simulink model "ITACG_3D_salvo_simulation"  (R2023b)
settings: Solver=ode4  StartTime=0.0  StopTime=28  FixedStep=1/10  RelTol=1e-3
libraries: simulink_extras x40, simulink x4
(part 2 of 2)

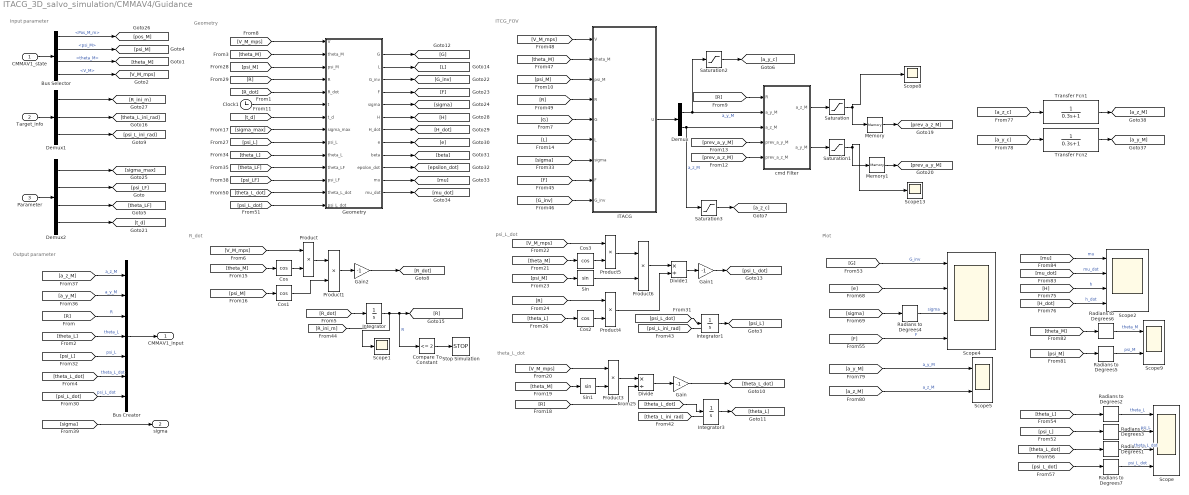
== system ITACG_3D_salvo_simulation/CMMAV4/Guidance ==
  note: Input parameter
  note: ITCG_FOV
  note: R_dot
  note: psi_L_dot
  note: theta_L_dot
  note: Output parameter
  note: Geometry
  note: Plot
  CMMAV1_state : Inport
  Target_info : Inport  Port=2
  Parameter : Inport  Port=3
  Bus Creator : BusCreator  Inputs=7
  Bus Selector : BusSelector  OutputSignals=Pos_M_m,psi_M,theta_M,V_M
  Clock1 : Clock
  Compare To Constant : simulink/Logic and Bit Operations/Compare To Constant  relop=<=  const=2  OutDataTypeStr=boolean
  Cos{,1..3} (4 alike) : Trigonometry  Operator=cos
  Demux : Demux  Outputs=2
  Demux1 : Demux  Outputs=3
  Demux2 : Demux
  Divide : Product  Inputs=*/
  Divide1 : Product  Inputs=*/
  Gain : Gain  Gain=-1
  Gain1 : Gain  Gain=-1
  Gain2 : Gain  Gain=-1
  Geometry : MATLAB Function  TreatAsAtomicUnit=on
  ITACG : MATLAB Function  TreatAsAtomicUnit=on
  Integrator : Integrator  InitialCondition=700
  Integrator1 : Integrator  InitialCondition=10*pi/180
  Integrator3 : Integrator  InitialCondition=-40*pi/180
  Memory : Memory
  Memory1 : Memory
  Product{,1,3..6} (6 alike) : Product
  Radians to Degrees{1..7} (7 alike) : simulink_extras/Transformations/Radians to Degrees
  Saturation{,1..3} (4 alike) : Saturate  UpperLimit=100  LowerLimit=-100
  Scope : Scope  NumInputPorts=4
  Scope1 : Scope
  Scope13 : Scope
  Scope2 : Scope  NumInputPorts=4
  Scope4 : Scope  NumInputPorts=4
  Scope5 : Scope  NumInputPorts=2
  Scope8 : Scope
  Scope9 : Scope  NumInputPorts=2
  Sin : Trigonometry
  Sin1 : Trigonometry
  Stop Simulation : Stop
  Transfer Fcn1 : TransferFcn  Denominator=[0.3 1]  ParameterTunability=Optimized
  Transfer Fcn2 : TransferFcn  Denominator=[0.3 1]  ParameterTunability=Optimized
  cmd Filter : MATLAB Function  TreatAsAtomicUnit=on
  CMMAV1_input : Outport
  sigma : Outport  Port=2
  wires:
  Product1/1 -> Gain2/1
  Gain2/1 -> [R_dot]
  [theta_L] -> Cos2/1
  [theta_L_dot] -> Integrator3/1
  Gain/1 -> [theta_L_dot]
  Product5/1 -> Product6/1
  Divide1/1 -> Gain1/1
  [V_M_mps] -> Product3/1
  [V_M_mps] -> Product5/1
  [theta_M] -> Sin1/1
  [R] -> Divide/2
  [theta_M] -> Cos3/1
  Divide/1 -> Gain/1
  [theta_M] -> Cos/1
  [R] -> Product4/1
  Product4/1 -> Divide1/2
  Integrator3/1 -> [theta_L]
  [psi_L_dot] -> Integrator1/1
  Sin1/1 -> Product3/2
  Product3/1 -> Divide/1
  [psi_M] -> Cos1/1
  Cos/1 -> Product/2
  Integrator1/1 -> [psi_L]
  Product6/1 -> Divide1/1
  [psi_M] -> Sin/1
  Compare To Constant/1 -> Stop Simulation/1
  [V_M_mps] -> Product/1
  Cos3/1 -> Product5/2
  Sin/1 -> Product6/2
  Integrator/1 -> Scope1/1, [R], Compare To Constant/1  "R"
  Product/1 -> Product1/1
  Cos2/1 -> Product4/2
  Cos1/1 -> Product1/2
  Gain1/1 -> [psi_L_dot]
  [R_dot] -> Integrator/1
  CMMAV1_state/1 -> Bus Selector/1
  Target_info/1 -> Demux1/1
  Demux2/1 -> [sigma_max]
  Parameter/1 -> Demux2/1
  Bus Selector/1 -> [pos_M]  "<Pos_M_m>"
  Bus Selector/4 -> [V_M_mps]  "<V_M>"
  Demux1/2 -> [theta_L_ini_rad]
  Demux1/3 -> [psi_L_ini_rad]
  Demux1/1 -> [R_ini_m]
  [psi_L] -> Bus Creator/5  "psi_L"
  [theta_L] -> Bus Creator/4  "theta_L"
  Bus Creator/1 -> CMMAV1_input/1
  [a_y_M] -> Bus Creator/2  "a_y_M"
  [R] -> Bus Creator/3  "R"
  [a_z_M] -> Bus Creator/1  "a_z_M"
  [theta_L_ini_rad] -> ?
  [psi_L_ini_rad] -> ?
  [R_ini_m] -> ?
  Bus Selector/2 -> [psi_M]  "<psi_M>"
  Bus Selector/3 -> [theta_M]  "<theta_M>"
  [psi_M] -> Geometry/3(psi_M)
  [V_M_mps] -> Geometry/1(V)
  [theta_M] -> Geometry/2(theta_M)
  [R] -> Geometry/4(R)
  Demux2/2 -> [psi_LF]
  Demux2/3 -> [theta_LF]
  Demux2/4 -> [t_d]
  Saturation2/1 -> [a_y_c]
  Saturation3/1 -> [a_z_c]
  cmd Filter/1(a_z_M) -> Saturation/1
  Memory/1 -> [prev_a_z_M]
  Transfer Fcn2/1 -> [a_y_M]
  Transfer Fcn1/1 -> [a_z_M]
  cmd Filter/2(a_y_M) -> Saturation1/1
  Saturation1/1 -> Scope13/1, Memory1/1
  Saturation/1 -> Scope8/1, Memory/1
  Demux/2 -> cmd Filter/3("a_z_M "), Saturation3/1  "a_z_M"
  [prev_a_y_M] -> cmd Filter/4(prev_a_y_M)
  [prev_a_z_M] -> cmd Filter/5(prev_a_z_M)
  [a_z_c] -> Transfer Fcn1/1
  Demux/1 -> cmd Filter/2("a_y_M "), Saturation2/1  "a_y_M"
  Memory1/1 -> [prev_a_y_M]
  [a_y_c] -> Transfer Fcn2/1
  [R] -> cmd Filter/1(R)
  ITACG/1(U) -> Demux/1
  [theta_LF] -> Geometry/11(theta_LF)
  [psi_LF] -> Geometry/12(psi_LF)
  [theta_L_dot] -> Geometry/13(theta_L_dot)
  [R_dot] -> Geometry/5(R_dot)
  [t_d] -> Geometry/7(t_d)
  [sigma_max] -> Geometry/8(sigma_max)
  [psi_L] -> Geometry/9(psi_L)
  [theta_L] -> Geometry/10(theta_L)
  [psi_L_dot] -> Geometry/14(psi_L_dot)
  Clock1/1 -> Geometry/6(t)
  Geometry/1(G) -> [G]
  Geometry/2(L) -> [L]
  Geometry/3(G_inv) -> [G_inv]
  Geometry/4(F) -> [F]
  Geometry/5(sigma) -> [sigma]
  Geometry/6(H) -> [H]
  Geometry/7(H_dot) -> [H_dot]
  Geometry/8(e) -> [e]
  Geometry/9(beta) -> [beta]
  Geometry/10(epsilon_dot) -> [epsilon_dot]
  Geometry/11(mu) -> [mu]
  Geometry/12(mu_dot) -> [mu_dot]
  [V_M_mps] -> ITACG/1(V)
  [theta_M] -> ITACG/2(theta_M)
  [psi_M] -> ITACG/3(psi_M)
  [G] -> ITACG/5(G)
  [L] -> ITACG/6(L)
  [sigma] -> ITACG/7(sigma)
  [F] -> ITACG/8(F)
  [G_inv] -> ITACG/9(G_inv)
  [R] -> ITACG/4(R)
  Radians to Degrees6/1 -> Scope9/1  "theta_M"
  Radians to Degrees7/1 -> Scope/4  "psi_L_dot"
  [psi_M] -> Radians to Degrees5/1
  [theta_L_dot] -> Radians to Degrees1/1
  Radians to Degrees3/1 -> Scope/2  "psi_L"
  [theta_L] -> Radians to Degrees2/1
  Radians to Degrees4/1 -> Scope4/3  "sigma"
  Radians to Degrees2/1 -> Scope/1  "theta_L"
  Radians to Degrees5/1 -> Scope9/2  "psi_M"
  [H] -> Scope2/3  "h"
  [psi_L] -> Radians to Degrees3/1
  [mu] -> Scope2/1  "mu"
  [mu_dot] -> Scope2/2  "mu_dot"
  Radians to Degrees1/1 -> Scope/3  "theta_L_dot"
  [sigma] -> Radians to Degrees4/1
  [a_y_M] -> Scope5/1  "a_y_M"
  [a_z_M] -> Scope5/2  "a_z_M"
  [G] -> Scope4/1  "G_inv"
  [theta_M] -> Radians to Degrees6/1
  [psi_L_dot] -> Radians to Degrees7/1
  [F] -> Scope4/4  "F"
  [H_dot] -> Scope2/4  "h_dot"
  [e] -> Scope4/2
  [theta_L_dot] -> Bus Creator/6  "theta_L_dot"
  [psi_L_dot] -> Bus Creator/7  "psi_L_dot"
  [sigma] -> sigma/1

== system ITACG_3D_salvo_simulation/CMMAV4/Parameter init ==
  Constant : Constant  Value=45
  Constant1 : Constant  Value=0
  Constant2 : Constant  Value=-80
  Constant3 : Constant  Value=28
  Degrees to Radians : simulink_extras/Transformations/Degrees to Radians
  Degrees to Radians1 : simulink_extras/Transformations/Degrees to Radians
  Degrees to Radians2 : simulink_extras/Transformations/Degrees to Radians
  Mux : Mux
  Parameter : Outport
  wires:
  Mux/1 -> Parameter/1
  Constant3/1 -> Mux/4  "t_d"
  Constant2/1 -> Degrees to Radians2/1
  Constant1/1 -> Degrees to Radians1/1
  Constant/1 -> Degrees to Radians/1
  Degrees to Radians2/1 -> Mux/3  "theta_LF"
  Degrees to Radians1/1 -> Mux/2  "psi_LF"
  Degrees to Radians/1 -> Mux/1  "sigma_max"

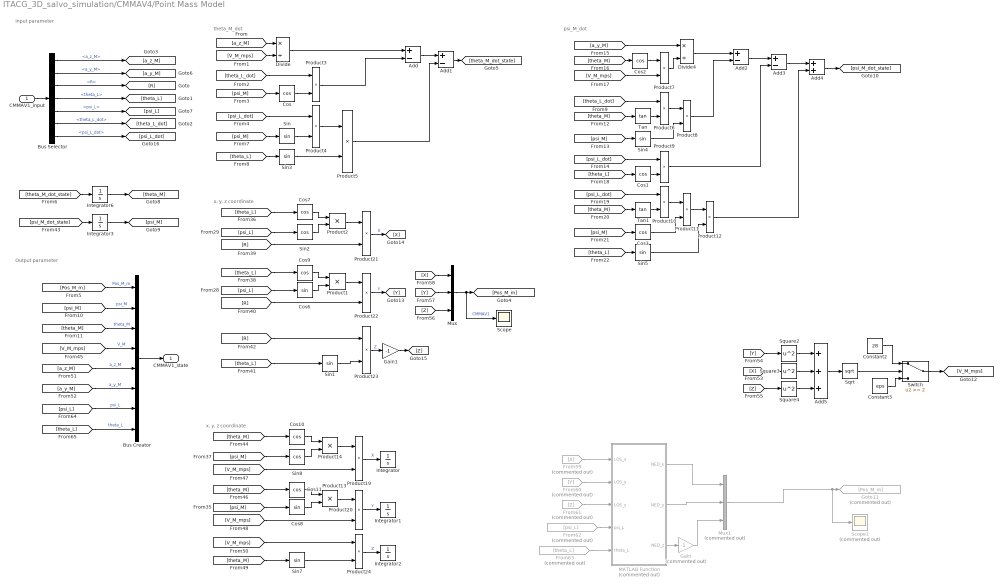
== system ITACG_3D_salvo_simulation/CMMAV4/Point Mass Model ==
  note: Input parameter
  note: x, y, z coordinate
  note: Output parameter
  note: x, y, z coordinate
  note: theta_M_dot
  note: psi_M_dot
  CMMAV1_input : Inport
  Add{,1..3} (4 alike) : Sum  Inputs=+-
  Add4 : Sum
  Add5 : Sum  Inputs=+++
  Bus Creator : BusCreator  Inputs=8
  Bus Selector : BusSelector  OutputSignals=a_z_M,a_y_M,R,theta_L,psi_L,theta_L_dot,psi_L_dot
  Constant2 : Constant  Value=28
  Constant3 : Constant  Value=eps
  Cos{,1..3,7,9..11} (8 alike) : Trigonometry  Operator=cos
  Cos6 : Trigonometry
  Cos8 : Trigonometry
  Divide : Product  Inputs=*/
  Divide4 : Product  Inputs=*/
  From59 : From  Commented=on  GotoTag=X
  From60 : From  Commented=on  GotoTag=Y
  From61 : From  Commented=on  GotoTag=Z
  From62 : From  Commented=on  GotoTag=psi_L
  From63 : From  Commented=on  GotoTag=theta_L
  Gain : Gain  Commented=on  Gain=-1
  Gain1 : Gain  Gain=-1
  Goto11 : Goto  Commented=on  GotoTag=Pos_M_m
  Integrator : Integrator
  Integrator1 : Integrator
  Integrator2 : Integrator
  Integrator3 : Integrator  InitialCondition=10*pi/180
  Integrator6 : Integrator  InitialCondition=10*pi/180
  MATLAB Function : MATLAB Function  Commented=on  TreatAsAtomicUnit=on
  Mux : Mux  Inputs=3
  Mux1 : Mux  Commented=on  Inputs=3
  Product{1..14,19..24} (20 alike) : Product
  Scope : Scope
  Scope1 : Scope  Commented=on
  Sin{,1,3..5,7} (6 alike) : Trigonometry
  Sin2 : Trigonometry  Operator=cos
  Sin8 : Trigonometry  Operator=cos
  Sqrt : Sqrt
  Square2 : Math  Operator=square
  Square3 : Math  Operator=square
  Square4 : Math  Operator=square
  Switch : Switch  Threshold=2  SaturateOnIntegerOverflow=off  InputSameDT=off
  Tan : Trigonometry  Operator=tan
  Tan1 : Trigonometry  Operator=tan
  CMMAV1_state : Outport
  wires:
  [psi_M] -> Bus Creator/2  "psi_M"
  [psi_M_dot_state] -> Integrator3/1
  [theta_L] -> Cos9/1
  [V_M_mps] -> Bus Creator/4  "V_M"
  Cos6/1 -> Product1/2
  Bus Selector/2 -> [a_y_M]  "<a_y_M>"
  Integrator6/1 -> [theta_M]
  [psi_L] -> Cos6/1
  Bus Selector/5 -> [psi_L]  "<psi_L>"
  Product21/1 -> [X]  "X"
  Product1/1 -> Product22/1
  Integrator3/1 -> [psi_M]
  Sin2/1 -> Product2/2
  Bus Selector/1 -> [a_z_M]  "<a_z_M>"
  Mux/1 -> [Pos_M_m], Scope/1  "CMMAV1"
  Bus Selector/3 -> [R]  "<R>"
  [theta_M] -> Bus Creator/3  "theta_M"
  [psi_L] -> Sin2/1
  Product2/1 -> Product21/1
  Cos9/1 -> Product1/1
  [theta_L] -> Cos7/1
  Cos7/1 -> Product2/1
  [theta_M_dot_state] -> Integrator6/1
  Product22/1 -> [Y]  "Y"
  [V_M_mps] -> Product24/1
  Sin7/1 -> Product24/2
  [V_M_mps] -> Product20/2
  [theta_M] -> Cos11/1
  [psi_M] -> Sin8/1
  [theta_M] -> Sin7/1
  Sin8/1 -> Product14/2
  Product14/1 -> Product19/1
  Product19/1 -> Integrator/1  "X"
  Product13/1 -> Product20/1
  Product24/1 -> Integrator2/1  "Z"
  [psi_M] -> Cos8/1
  [V_M_mps] -> Product19/2
  [theta_M] -> Cos10/1
  Cos11/1 -> Product13/1
  Cos8/1 -> Product13/2
  Product20/1 -> Integrator1/1  "Y"
  Cos10/1 -> Product14/1
  [R] -> Product21/2
  [R] -> Product22/2
  [R] -> Product23/1
  Sin1/1 -> Product23/2
  [theta_L] -> Sin1/1
  CMMAV1_input/1 -> Bus Selector/1
  [Pos_M_m] -> Bus Creator/1  "Pos_M_m"
  Bus Creator/1 -> CMMAV1_state/1
  Bus Selector/4 -> [theta_L]  "<theta_L>"
  [a_z_M] -> Bus Creator/5  "a_z_M"
  [a_y_M] -> Bus Creator/6  "a_y_M"
  Constant3/1 -> Switch/3
  Switch/1 -> [V_M_mps]
  Sqrt/1 -> Switch/2
  Add5/1 -> Sqrt/1
  Square2/1 -> Add5/1
  [Y] -> Square2/1
  Constant2/1 -> Switch/1
  [X] -> Square3/1
  Square3/1 -> Add5/2
  Product23/1 -> Gain1/1  "Z"
  [Z] -> Square4/1
  [X] -> Mux/1
  [Y] -> Mux/2
  [Z] -> Mux/3
  Square4/1 -> Add5/3
  From59/1 -> MATLAB Function/1(LOS_x)
  From60/1 -> MATLAB Function/2(LOS_y)
  From61/1 -> MATLAB Function/3(LOS_z)
  From62/1 -> MATLAB Function/4(psi_L)
  From63/1 -> MATLAB Function/5(theta_L)
  MATLAB Function/2(NED_y) -> Mux1/2
  MATLAB Function/1(NED_x) -> Mux1/1
  MATLAB Function/3(NED_z) -> Gain/1
  Gain/1 -> Mux1/3
  Mux1/1 -> Scope1/1, Goto11/1
  [psi_L] -> Bus Creator/7  "psi_L"
  [theta_L] -> Bus Creator/8  "theta_L"
  Product5/1 -> Add1/2
  Add/1 -> Add1/1
  Product4/1 -> Product5/1
  [a_z_M] -> Divide/1
  Divide/1 -> Add/1
  [V_M_mps] -> Divide/2
  Sin3/1 -> Product5/2
  Sin/1 -> Product4/2
  [psi_L_dot] -> Product4/1
  [psi_M] -> Cos/1
  Cos/1 -> Product3/2
  Add1/1 -> [theta_M_dot_state]
  Product3/1 -> Add/2
  [psi_M] -> Sin/1
  [theta_L] -> Sin3/1
  [theta_L_dot] -> Product3/1
  Product8/1 -> Add2/2
  [a_y_M] -> Divide4/1
  Product7/1 -> Divide4/2
  Divide4/1 -> Add2/1
  [V_M_mps] -> Product7/2
  Product6/1 -> Product8/1
  Product10/1 -> Product11/1
  Tan1/1 -> Product10/2
  [theta_L] -> Cos1/1
  Product12/1 -> Add4/2
  [theta_L] -> Sin5/1
  Product11/1 -> Product12/1
  [theta_L_dot] -> Product6/1
  Sin5/1 -> Product12/2
  Cos3/1 -> Product11/2
  [psi_M] -> Cos3/1
  Product9/1 -> Add3/2
  Add4/1 -> [psi_M_dot_state]
  [psi_L_dot] -> Product10/1
  [theta_M] -> Tan1/1
  Cos1/1 -> Product9/2
  [theta_M] -> Cos2/1
  Sin4/1 -> Product8/2
  [psi_M] -> Sin4/1
  [theta_M] -> Tan/1
  Tan/1 -> Product6/2
  [psi_L_dot] -> Product9/1
  Cos2/1 -> Product7/1
  Add2/1 -> Add3/1
  Add3/1 -> Add4/1
  Gain1/1 -> [Z]
  Bus Selector/6 -> [theta_L_dot]  "<theta_L_dot>"
  Bus Selector/7 -> [psi_L_dot]  "<psi_L_dot>"

== system ITACG_3D_salvo_simulation/CMMAV4/Target ==
  note: LOS_angle initial
  note: Target position
  note: Target parameter
  note: Output parameter
  note: R_initial
  note: Output parameter
  Add : Sum
  Add1 : Sum
  Add2 : Sum
  Asin : Trigonometry  Operator=asin
  Asin1 : Trigonometry  Operator=acos
  Demux : Demux  Outputs=3
  Demux1 : Demux  Outputs=3
  Divide : Product  Inputs=*/
  Divide1 : Product  Inputs=*/
  Integrator : Integrator
  Integrator1 : Integrator
  Integrator2 : Integrator
  Mux : Mux  Inputs=3
  Mux1 : Mux  Inputs=3
  Scope : Scope
  Sqrt : Sqrt
  Sqrt1 : Sqrt
  Square{1..5} (5 alike) : Math  Operator=square
  Sum : Sum  Inputs=+++
  Sum1 : Sum  Inputs=++|
  Target Position : Constant  Value=[300;-500;300]  VectorParams1D=off
  Target Velocity : Constant  Value=[0;0;0]  VectorParams1D=off
  Target_info : Outport
  wires:
  [psi_L_ini_rad] -> Mux/3
  Asin/1 -> [theta_L_ini_rad]
  [rT_ini_z_m] -> Mux1/3
  [rM_z] -> Add2/1
  Demux/3 -> [vT_z]
  [vT_z] -> Integrator2/1
  Demux/2 -> [vT_y]
  [rT_ini_x_m] -> Mux1/1
  Add1/1 -> [rT_ini_y_m]  "Y"
  Square2/1 -> Sum/1
  [vT_x] -> Integrator/1
  Mux1/1 -> [Pos_T_m]
  Square3/1 -> Sum/2
  Add2/1 -> [rT_ini_z_m]  "Z"
  Integrator/1 -> [vT_xt]
  Sum/1 -> Sqrt/1
  Demux1/3 -> [rM_z]
  [rT_ini_y_m] -> Mux1/2
  Integrator1/1 -> [vT_yt]
  Demux/1 -> [vT_x]
  Demux1/1 -> [rM_x]
  Target Velocity/1 -> Demux/1
  Demux1/2 -> [rM_y]
  Add/1 -> [rT_ini_x_m]  "X"
  [vT_yt] -> Add1/2
  Divide1/1 -> Asin1/1
  [rM_x] -> Add/1
  [vT_zt] -> Add2/2
  Sum1/1 -> Sqrt1/1
  [rT_ini_x_m] -> Square1/1
  Square1/1 -> Sum1/1
  Square5/1 -> Sum1/2
  [rT_ini_y_m] -> Square5/1
  [vT_y] -> Integrator1/1
  [rM_y] -> Add1/1
  [rT_ini_z_m] -> Divide/1
  [R_ini_m] -> Mux/1
  Sqrt/1 -> Scope/1, [R_ini_m]
  [R_ini_m] -> Divide/2
  [rT_ini_z_m] -> Square4/1
  Sqrt1/1 -> Divide1/2
  [vT_xt] -> Add/2
  Divide/1 -> Asin/1
  Integrator2/1 -> [vT_zt]
  Square4/1 -> Sum/3
  [rT_ini_x_m] -> Divide1/1
  [theta_L_ini_rad] -> Mux/2
  Asin1/1 -> [psi_L_ini_rad]
  Mux/1 -> Target_info/1
  Target Position/1 -> Demux1/1
  [rT_ini_y_m] -> Square3/1
  [rT_ini_x_m] -> Square2/1

== matlab function ITACG_3D_salvo_simulation/CMMAV1/Guidance/ITACG ==
  data: U output; V input; theta_M input; psi_M input; R input; G input; L input; sigma input; F input; G_inv input
function U  = fcn(V, theta_M, psi_M, R, G, L, sigma, F, G_inv)
    D2R = 180/pi;
    N=4;
    sigma_s = 0.001 * D2R;
    % sigma_deg = sigma*180/pi;
    U_PN = [-sin(psi_M) -sin(theta_M)*cos(psi_M)]';
    %% G_inv
    % U_eq = G_inv * F;

    % if abs(sigma) > sigma_s
    %     U = G_inv * L + U_eq;
    % else
    %     U = N * V^2 * U_PN / R;
    % end
    % U = G_inv * L + U_eq;

    %% G^-1
    U_eq = G^-1 * F;

    if abs(sigma) > sigma_s
        U = G^-1 * L - U_eq;
    else
        U = N * V^2 * U_PN / R;
    end

== matlab function ITACG_3D_salvo_simulation/CMMAV1/Guidance/Geometry ==
  data: V input; theta_M input; psi_M input; R input; R_dot input; G output; L output; t input; t_d input; sigma_max input; psi_L input; theta_L input; theta_LF input; psi_LF input; theta_L_dot input; psi_L_dot input; G_inv output; F output; sigma output; H output; H_dot output; e output; beta output; epsilon_dot output; mu output; mu_dot output
function [G, L, G_inv, F, sigma, H, H_dot, e, beta, epsilon_dot, mu, mu_dot] =fcn(V, theta_M, psi_M, R, R_dot, t, t_d, sigma_max, psi_L, theta_L, theta_LF, psi_LF, theta_L_dot, psi_L_dot)
    %% constant parameter
    b= 0.1;
    k= 1.4;
    eta = 0.5;
    T_s = 0.6 * t_d;

    %% guidance parameter
    sigma = acos(cos(theta_M) * cos(psi_M));
    t_go = t_d - t;

    %% epsilon
    epsilon = t_go - R / V;
    epsilon_dot = cos(sigma) - 1;

    %% theta_e
    theta_e = theta_L - theta_LF;
    theta_e_dot = theta_L_dot;

    %% psi_e
    psi_e = psi_L - psi_LF;
    psi_e_dot = psi_L_dot;

    %% beta
    beta = (theta_e^2 + cos(theta_L)^2 * psi_e^2) / (4 * V^2);
    % beta = sin(sigma)^2 * theta_e / (4 * V^2 * sin(theta_M)^2);

    beta_dot = (theta_e * theta_e_dot + cos(theta_L)^2 * psi_e * psi_e_dot - sin(theta_L) * cos(theta_L) * psi_e^2 * theta_L_dot) / (2 * V^2);

    %% C_f/C_g  
    C_f = psi_e * sin(theta_L) * cos(theta_L);
    C_g = psi_e * cos(theta_M) * cos(theta_L) + theta_e * sin(theta_M) * sin(psi_M);

    %% H
    H = (2 * epsilon^2) / (beta * R^2 + epsilon^2);
    H_dot = ((4 * epsilon * epsilon_dot) / (beta * R^2 + epsilon^2)) - ((2 * epsilon^2 * (beta_dot * R^2 + 2 * beta * R * R_dot + 2 * epsilon * epsilon_dot)) / (beta * R^2 + epsilon^2)^2);
    H_max = 1 - cos(sigma_max);
    H_bar = H / H_max;

    %% chi
    if abs(theta_L) >= pi/2
        chi = theta_e * sin(theta_M);
    else
        chi = psi_e * cos(theta_M) * cos(theta_L) * sin(psi_M) + theta_e * sin(theta_M);
    end
    %% F(H)
    if H < eta * H_max
        f_h = H;
    else
        f_h = ((1 - eta) * tanh((H_bar - eta) / (1 - eta)) + eta) * H_max;
    end
    %% F(H)_dot
    if H < eta * H_max
        f_h_dot = H_dot;
    else
        f_h_dot = (1 - tanh((H_bar - eta) / (1 - eta))^2) * H_dot;
    end

    %% mu    
    if t >= 0 && t < T_s
        mu = T_s / (T_s - t);
        mu_dot = T_s / (T_s - t)^2;
    else
        mu = 1;
        mu_dot = 0;
    end

    %% Baseline Error Dynamics
    % e = [epsilon_dot + H;
    %     psi_e * theta_e_dot - theta_e * psi_e_dot];
    % 
    % F = [-R * theta_L_dot^2 / V - R * psi_L_dot^2 * cos(theta_L)^2 / V + H_dot;
    %     2 * (theta_e * psi_L_dot - psi_e * theta_L_dot) * R_dot / R - C_f * psi_L_dot^2 - 2 * theta_e * psi_L_dot * theta_L_dot * tan(theta_L)]; 

    %% Nonlinear Error Dynamics
    e = [epsilon_dot + f_h;
        psi_e * theta_e_dot - theta_e * psi_e_dot];

    F = [-R * theta_L_dot^2 / V - R * psi_L_dot^2 * cos(theta_L)^2 / V + f_h_dot;
        2 * (theta_e * psi_L_dot - psi_e * theta_L_dot) * R_dot / R - C_f * psi_L_dot^2 - 2 * theta_e * psi_L_dot * theta_L_dot * tan(theta_L)]; 

    %% guidance vector
    G = [-sin(psi_M) / V, -sin(theta_M) * cos(psi_M) / V;
        theta_e * cos(psi_M) / (R * cos(theta_L)), -C_g / (R * cos(theta_L))];

    G_inv = 1 / chi * [-V * C_g, R * sin(theta_M) * cos(psi_M) * cos(theta_L);
        -V * theta_e * cos(psi_M), -R * sin(psi_M) * cos(theta_L)];

    % ne = norm(e);
    L = -(b + k * mu_dot / mu) * e;

== matlab function ITACG_3D_salvo_simulation/CMMAV2/Guidance/ITACG ==
  data: U output; V input; theta_M input; psi_M input; R input; G input; L input; sigma input; F input; G_inv input
function U  = fcn(V, theta_M, psi_M, R, G, L, sigma, F, G_inv)
    D2R = 180/pi;
    N=4;
    sigma_s = 0.001 * D2R;
    % sigma_deg = sigma*180/pi;
    U_PN = [-sin(psi_M) -sin(theta_M)*cos(psi_M)]';
    %% G_inv
    % U_eq = G_inv * F;

    % if abs(sigma) > sigma_s
    %     U = G_inv * L + U_eq;
    % else
    %     U = N * V^2 * U_PN / R;
    % end
    % U = G_inv * L + U_eq;

    %% G^-1
    U_eq = G^-1 * F;

    if abs(sigma) > sigma_s
        U = G^-1 * L - U_eq;
    else
        U = N * V^2 * U_PN / R;
    end

== matlab function ITACG_3D_salvo_simulation/CMMAV2/Guidance/cmd Filter ==
  data: R input; a_y_M input; a_z_M output; a_z_M input; prev_a_y_M input; prev_a_z_M input; a_y_M output
function [a_z_M, a_y_M] = fcn(R, a_y_M, a_z_M, prev_a_y_M, prev_a_z_M)

if R<10
    a_z_M = prev_a_z_M;
    a_y_M = prev_a_y_M;
end

== matlab function ITACG_3D_salvo_simulation/CMMAV2/Point Mass Model/MATLAB Function ==
  data: LOS_x input; NED_x output; LOS_y input; LOS_z input; psi_L input; theta_L input; NED_y output; NED_z output
function [NED_x, NED_y, NED_z] = fcn(LOS_x, LOS_y, LOS_z, psi_L, theta_L)

% 입력 벡터 (LOS 기준)
v_LOS = [LOS_x; LOS_y; LOS_z];

% 1. LOS → RCS 회전행렬 (T_LOS_to_RCS)
Rz_psi = [cos(psi_L),  sin(psi_L), 0;
         -sin(psi_L),  cos(psi_L), 0;
          0,           0,          1];

Ry_theta = [cos(theta_L), 0, -sin(theta_L);
            0,           1,  0;
            sin(theta_L), 0,  cos(theta_L)];

T_LOS_to_RCS = Ry_theta * Rz_psi;

% 2. RCS → NED 변환 (Z축 반전만 적용)
T_RCS_to_NED = [1, 0,  0;
                0, 1,  0;
                0, 0, -1];

% 전체 변환: LOS → RCS → NED
T_total = T_RCS_to_NED * T_LOS_to_RCS;

v_NED = T_total * v_LOS;

% 결과 추출
NED_x = v_NED(1);
NED_y = v_NED(2);
NED_z = v_NED(3);

end

== matlab function ITACG_3D_salvo_simulation/CMMAV3/Guidance/Geometry ==
  data: V input; theta_M input; psi_M input; R input; R_dot input; G output; L output; t input; t_d input; sigma_max input; psi_L input; theta_L input; theta_LF input; psi_LF input; theta_L_dot input; psi_L_dot input; G_inv output; F output; sigma output; H output; H_dot output; e output; beta output; epsilon_dot output; mu output; mu_dot output
function [G, L, G_inv, F, sigma, H, H_dot, e, beta, epsilon_dot, mu, mu_dot] =fcn(V, theta_M, psi_M, R, R_dot, t, t_d, sigma_max, psi_L, theta_L, theta_LF, psi_LF, theta_L_dot, psi_L_dot)
    %% constant parameter
    b= 0.1;
    k= 1.4;
    eta = 0.5;
    T_s = 0.6 * t_d;

    %% guidance parameter
    sigma = acos(cos(theta_M) * cos(psi_M));
    t_go = t_d - t;

    %% epsilon
    epsilon = t_go - R / V;
    epsilon_dot = cos(sigma) - 1;

    %% theta_e
    theta_e = theta_L - theta_LF;
    theta_e_dot = theta_L_dot;

    %% psi_e
    psi_e = psi_L - psi_LF;
    psi_e_dot = psi_L_dot;

    %% beta
    beta = (theta_e^2 + cos(theta_L)^2 * psi_e^2) / (4 * V^2);
    % beta = sin(sigma)^2 * theta_e / (4 * V^2 * sin(theta_M)^2);

    beta_dot = (theta_e * theta_e_dot + cos(theta_L)^2 * psi_e * psi_e_dot - sin(theta_L) * cos(theta_L) * psi_e^2 * theta_L_dot) / (2 * V^2);

    %% C_f/C_g  
    C_f = psi_e * sin(theta_L) * cos(theta_L);
    C_g = psi_e * cos(theta_M) * cos(theta_L) + theta_e * sin(theta_M) * sin(psi_M);

    %% H
    H = (2 * epsilon^2) / (beta * R^2 + epsilon^2);
    H_dot = ((4 * epsilon * epsilon_dot) / (beta * R^2 + epsilon^2)) - ((2 * epsilon^2 * (beta_dot * R^2 + 2 * beta * R * R_dot + 2 * epsilon * epsilon_dot)) / (beta * R^2 + epsilon^2)^2);
    H_max = 1 - cos(sigma_max);
    H_bar = H / H_max;

    %% chi
    if abs(theta_L) >= pi/2
        chi = theta_e * sin(theta_M);
    else
        chi = psi_e * cos(theta_M) * cos(theta_L) * sin(psi_M) + theta_e * sin(theta_M);
    end
    %% F(H)
    if H < eta * H_max
        f_h = H;
    else
        f_h = ((1 - eta) * tanh((H_bar - eta) / (1 - eta)) + eta) * H_max;
    end
    %% F(H)_dot
    if H < eta * H_max
        f_h_dot = H_dot;
    else
        f_h_dot = (1 - tanh((H_bar - eta) / (1 - eta))^2) * H_dot;
    end

    %% mu    
    if t >= 0 && t < T_s
        mu = T_s / (T_s - t);
        mu_dot = T_s / (T_s - t)^2;
    else
        mu = 1;
        mu_dot = 0;
    end

    %% Baseline Error Dynamics
    % e = [epsilon_dot + H;
    %     psi_e * theta_e_dot - theta_e * psi_e_dot];
    % 
    % F = [-R * theta_L_dot^2 / V - R * psi_L_dot^2 * cos(theta_L)^2 / V + H_dot;
    %     2 * (theta_e * psi_L_dot - psi_e * theta_L_dot) * R_dot / R - C_f * psi_L_dot^2 - 2 * theta_e * psi_L_dot * theta_L_dot * tan(theta_L)]; 

    %% Nonlinear Error Dynamics
    e = [epsilon_dot + f_h;
        psi_e * theta_e_dot - theta_e * psi_e_dot];

    F = [-R * theta_L_dot^2 / V - R * psi_L_dot^2 * cos(theta_L)^2 / V + f_h_dot;
        2 * (theta_e * psi_L_dot - psi_e * theta_L_dot) * R_dot / R - C_f * psi_L_dot^2 - 2 * theta_e * psi_L_dot * theta_L_dot * tan(theta_L)]; 

    %% guidance vector
    G = [-sin(psi_M) / V, -sin(theta_M) * cos(psi_M) / V;
        theta_e * cos(psi_M) / (R * cos(theta_L)), -C_g / (R * cos(theta_L))];

    G_inv = 1 / chi * [-V * C_g, R * sin(theta_M) * cos(psi_M) * cos(theta_L);
        -V * theta_e * cos(psi_M), -R * sin(psi_M) * cos(theta_L)];

    % ne = norm(e);
    L = -(b + k * mu_dot / mu) * e;

== matlab function ITACG_3D_salvo_simulation/CMMAV3/Guidance/ITACG ==
  data: U output; V input; theta_M input; psi_M input; R input; G input; L input; sigma input; F input; G_inv input
function U  = fcn(V, theta_M, psi_M, R, G, L, sigma, F, G_inv)
    D2R = 180/pi;
    N=4;
    sigma_s = 0.001 * D2R;
    % sigma_deg = sigma*180/pi;
    U_PN = [-sin(psi_M) -sin(theta_M)*cos(psi_M)]';
    %% G_inv
    % U_eq = G_inv * F;

    % if abs(sigma) > sigma_s
    %     U = G_inv * L + U_eq;
    % else
    %     U = N * V^2 * U_PN / R;
    % end
    % U = G_inv * L + U_eq;

    %% G^-1
    U_eq = G^-1 * F;

    if abs(sigma) > sigma_s
        U = G^-1 * L - U_eq;
    else
        U = N * V^2 * U_PN / R;
    end

== matlab function ITACG_3D_salvo_simulation/CMMAV3/Guidance/cmd Filter ==
  data: R input; a_y_M input; a_z_M output; a_z_M input; prev_a_y_M input; prev_a_z_M input; a_y_M output
function [a_z_M, a_y_M] = fcn(R, a_y_M, a_z_M, prev_a_y_M, prev_a_z_M)

if R<10
    a_z_M = prev_a_z_M;
    a_y_M = prev_a_y_M;
end

== matlab function ITACG_3D_salvo_simulation/CMMAV3/Point Mass Model/MATLAB Function ==
  data: LOS_x input; NED_x output; LOS_y input; LOS_z input; psi_L input; theta_L input; NED_y output; NED_z output
function [NED_x, NED_y, NED_z] = fcn(LOS_x, LOS_y, LOS_z, psi_L, theta_L)

% 입력 벡터 (LOS 기준)
v_LOS = [LOS_x; LOS_y; LOS_z];

% 1. LOS → RCS 회전행렬 (T_LOS_to_RCS)
Rz_psi = [cos(psi_L),  sin(psi_L), 0;
         -sin(psi_L),  cos(psi_L), 0;
          0,           0,          1];

Ry_theta = [cos(theta_L), 0, -sin(theta_L);
            0,           1,  0;
            sin(theta_L), 0,  cos(theta_L)];

T_LOS_to_RCS = Ry_theta * Rz_psi;

% 2. RCS → NED 변환 (Z축 반전만 적용)
T_RCS_to_NED = [1, 0,  0;
                0, 1,  0;
                0, 0, -1];

% 전체 변환: LOS → RCS → NED
T_total = T_RCS_to_NED * T_LOS_to_RCS;

v_NED = T_total * v_LOS;

% 결과 추출
NED_x = v_NED(1);
NED_y = v_NED(2);
NED_z = v_NED(3);

end

== matlab function ITACG_3D_salvo_simulation/CMMAV4/Guidance/Geometry ==
  data: V input; theta_M input; psi_M input; R input; R_dot input; G output; L output; t input; t_d input; sigma_max input; psi_L input; theta_L input; theta_LF input; psi_LF input; theta_L_dot input; psi_L_dot input; G_inv output; F output; sigma output; H output; H_dot output; e output; beta output; epsilon_dot output; mu output; mu_dot output
function [G, L, G_inv, F, sigma, H, H_dot, e, beta, epsilon_dot, mu, mu_dot] =fcn(V, theta_M, psi_M, R, R_dot, t, t_d, sigma_max, psi_L, theta_L, theta_LF, psi_LF, theta_L_dot, psi_L_dot)
    %% constant parameter
    b= 0.1;
    k= 1.4;
    eta = 0.5;
    T_s = 0.6 * t_d;

    %% guidance parameter
    sigma = acos(cos(theta_M) * cos(psi_M));
    t_go = t_d - t;

    %% epsilon
    epsilon = t_go - R / V;
    epsilon_dot = cos(sigma) - 1;

    %% theta_e
    theta_e = theta_L - theta_LF;
    theta_e_dot = theta_L_dot;

    %% psi_e
    psi_e = psi_L - psi_LF;
    psi_e_dot = psi_L_dot;

    %% beta
    beta = (theta_e^2 + cos(theta_L)^2 * psi_e^2) / (4 * V^2);
    % beta = sin(sigma)^2 * theta_e / (4 * V^2 * sin(theta_M)^2);

    beta_dot = (theta_e * theta_e_dot + cos(theta_L)^2 * psi_e * psi_e_dot - sin(theta_L) * cos(theta_L) * psi_e^2 * theta_L_dot) / (2 * V^2);

    %% C_f/C_g  
    C_f = psi_e * sin(theta_L) * cos(theta_L);
    C_g = psi_e * cos(theta_M) * cos(theta_L) + theta_e * sin(theta_M) * sin(psi_M);

    %% H
    H = (2 * epsilon^2) / (beta * R^2 + epsilon^2);
    H_dot = ((4 * epsilon * epsilon_dot) / (beta * R^2 + epsilon^2)) - ((2 * epsilon^2 * (beta_dot * R^2 + 2 * beta * R * R_dot + 2 * epsilon * epsilon_dot)) / (beta * R^2 + epsilon^2)^2);
    H_max = 1 - cos(sigma_max);
    H_bar = H / H_max;

    %% chi
    if abs(theta_L) >= pi/2
        chi = theta_e * sin(theta_M);
    else
        chi = psi_e * cos(theta_M) * cos(theta_L) * sin(psi_M) + theta_e * sin(theta_M);
    end
    %% F(H)
    if H < eta * H_max
        f_h = H;
    else
        f_h = ((1 - eta) * tanh((H_bar - eta) / (1 - eta)) + eta) * H_max;
    end
    %% F(H)_dot
    if H < eta * H_max
        f_h_dot = H_dot;
    else
        f_h_dot = (1 - tanh((H_bar - eta) / (1 - eta))^2) * H_dot;
    end

    %% mu    
    if t >= 0 && t < T_s
        mu = T_s / (T_s - t);
        mu_dot = T_s / (T_s - t)^2;
    else
        mu = 1;
        mu_dot = 0;
    end

    %% Baseline Error Dynamics
    % e = [epsilon_dot + H;
    %     psi_e * theta_e_dot - theta_e * psi_e_dot];
    % 
    % F = [-R * theta_L_dot^2 / V - R * psi_L_dot^2 * cos(theta_L)^2 / V + H_dot;
    %     2 * (theta_e * psi_L_dot - psi_e * theta_L_dot) * R_dot / R - C_f * psi_L_dot^2 - 2 * theta_e * psi_L_dot * theta_L_dot * tan(theta_L)]; 

    %% Nonlinear Error Dynamics
    e = [epsilon_dot + f_h;
        psi_e * theta_e_dot - theta_e * psi_e_dot];

    F = [-R * theta_L_dot^2 / V - R * psi_L_dot^2 * cos(theta_L)^2 / V + f_h_dot;
        2 * (theta_e * psi_L_dot - psi_e * theta_L_dot) * R_dot / R - C_f * psi_L_dot^2 - 2 * theta_e * psi_L_dot * theta_L_dot * tan(theta_L)]; 

    %% guidance vector
    G = [-sin(psi_M) / V, -sin(theta_M) * cos(psi_M) / V;
        theta_e * cos(psi_M) / (R * cos(theta_L)), -C_g / (R * cos(theta_L))];

    G_inv = 1 / chi * [-V * C_g, R * sin(theta_M) * cos(psi_M) * cos(theta_L);
        -V * theta_e * cos(psi_M), -R * sin(psi_M) * cos(theta_L)];

    % ne = norm(e);
    L = -(b + k * mu_dot / mu) * e;

== matlab function ITACG_3D_salvo_simulation/CMMAV1/Point Mass Model/MATLAB Function ==
  data: LOS_x input; NED_x output; LOS_y input; LOS_z input; psi_L input; theta_L input; NED_y output; NED_z output
function [NED_x, NED_y, NED_z] = fcn(LOS_x, LOS_y, LOS_z, psi_L, theta_L)

% 입력 벡터 (LOS 기준)
v_LOS = [LOS_x; LOS_y; LOS_z];

% 1. LOS → RCS 회전행렬 (T_LOS_to_RCS)
Rz_psi = [cos(psi_L),  sin(psi_L), 0;
         -sin(psi_L),  cos(psi_L), 0;
          0,           0,          1];

Ry_theta = [cos(theta_L), 0, -sin(theta_L);
            0,           1,  0;
            sin(theta_L), 0,  cos(theta_L)];

T_LOS_to_RCS = Ry_theta * Rz_psi;

% 2. RCS → NED 변환 (Z축 반전만 적용)
T_RCS_to_NED = [1, 0,  0;
                0, 1,  0;
                0, 0, -1];

% 전체 변환: LOS → RCS → NED
T_total = T_RCS_to_NED * T_LOS_to_RCS;

v_NED = T_total * v_LOS;

% 결과 추출
NED_x = v_NED(1);
NED_y = v_NED(2);
NED_z = v_NED(3);

end

== matlab function ITACG_3D_salvo_simulation/Figure/MATLAB Function ==
  settings: updateMethod=DISCRETE
  data: CMMAV1_x input; CMMAV1_y input; CMMAV1_z input; CMMAV2_x input; CMMAV2_y input; CMMAV2_z input; CMMAV3_x input; CMMAV3_y input; CMMAV3_z input; CMMAV4_x input; CMMAV4_y input; CMMAV4_z input
function fcn(CMMAV1_x, CMMAV1_y, CMMAV1_z, CMMAV2_x, CMMAV2_y, CMMAV2_z, CMMAV3_x, CMMAV3_y, CMMAV3_z, CMMAV4_x, CMMAV4_y, CMMAV4_z)

persistent timeldx data1 data2 data3 data4 d12_hist d13_hist d14_hist d23_hist d24_hist d34_hist

if isempty(data1)
    data1=zeros(100000,3); data2=zeros(100000,3);
    data3=zeros(100000,3); data4=zeros(100000,3);
    d12_hist = zeros(100000,1); d13_hist = zeros(100000,1); d14_hist = zeros(100000,1);
    d23_hist = zeros(100000,1); d24_hist = zeros(100000,1); d34_hist = zeros(100000,1);
    timeldx=1;
end

% 위치 저장
CMMAV1 = [CMMAV1_x, CMMAV1_y, CMMAV1_z];
CMMAV2 = [CMMAV2_x, CMMAV2_y, CMMAV2_z];
CMMAV3 = [CMMAV3_x, CMMAV3_y, CMMAV3_z];
CMMAV4 = [CMMAV4_x, CMMAV4_y, CMMAV4_z];

data1(timeldx, :) = CMMAV1;
data2(timeldx, :) = CMMAV2;
data3(timeldx, :) = CMMAV3;
data4(timeldx, :) = CMMAV4;

% 상대 거리 계산
d12_hist(timeldx) = norm(CMMAV1 - CMMAV2);
d13_hist(timeldx) = norm(CMMAV1 - CMMAV3);
d14_hist(timeldx) = norm(CMMAV1 - CMMAV4);
d23_hist(timeldx) = norm(CMMAV2 - CMMAV3);
d24_hist(timeldx) = norm(CMMAV2 - CMMAV4);
d34_hist(timeldx) = norm(CMMAV3 - CMMAV4);

% === Figure 1: 3D Trajectory ===
figure(1); clf; 
grid on; hold on; axis equal; view(3); box on;
plot3(data1(1:timeldx,1), data1(1:timeldx,2), data1(1:timeldx,3), 'r', 'LineWidth', 1.5);
plot3(data2(1:timeldx,1), data2(1:timeldx,2), data2(1:timeldx,3), 'b', 'LineWidth', 1.5);
plot3(data3(1:timeldx,1), data3(1:timeldx,2), data3(1:timeldx,3), 'g', 'LineWidth', 1.5);
plot3(data4(1:timeldx,1), data4(1:timeldx,2), data4(1:timeldx,3), 'm', 'LineWidth', 1.5);
scatter3(0, 0, 0, 100, 'k', 'o', 'filled');
scatter3(CMMAV1_x, CMMAV1_y, CMMAV1_z, 100, 'r', 's', 'filled');
scatter3(CMMAV2_x, CMMAV2_y, CMMAV2_z, 100, 'b', 'd', 'filled');
scatter3(CMMAV3_x, CMMAV3_y, CMMAV3_z, 100, 'g', '^', 'filled');
scatter3(CMMAV4_x, CMMAV4_y, CMMAV4_z, 100, 'm', 'p', 'filled');
legend({'UAV1','UAV2','UAV3','UAV4'}, 'Location', 'best', 'FontSize', 16, 'FontWeight', 'bold', 'FontAngle', 'italic');
xlabel('X (m)', 'FontSize', 16, 'FontWeight', 'bold', 'FontAngle', 'italic'); 
ylabel('Y (m)', 'FontSize', 16, 'FontWeight', 'bold', 'FontAngle', 'italic'); 
zlabel('Z (m)', 'FontSize', 16, 'FontWeight', 'bold', 'FontAngle', 'italic');
% xlim([-100 400]); ylim([-100 600]); zlim([0 400]);
set(gca, 'FontSize', 16, ...
         ...
         'FontAngle', 'italic', ...
         'FontName', 'Times New Roman');

% 
% % === Figure 2: Relative Distance ===
% figure(2); clf;
% hold on;
% box on;
% t_vec = 0.1 * (0:timeldx-1); 
% 
% % --- 상대거리 선들 ---
% plot(t_vec, d12_hist(1:timeldx), 'r', 'LineWidth', 1.2);
% plot(t_vec, d13_hist(1:timeldx), 'g', 'LineWidth', 1.2);
% plot(t_vec, d14_hist(1:timeldx), 'b', 'LineWidth', 1.2);
% plot(t_vec, d23_hist(1:timeldx), 'c', 'LineWidth', 1.2);
% plot(t_vec, d24_hist(1:timeldx), 'm', 'LineWidth', 1.2);
% plot(t_vec, d34_hist(1:timeldx), 'k', 'LineWidth', 1.2);
% 
% % --- d_safety 선만 plot하고 핸들 저장 ---
% h = plot([0, 350], [10, 10], 'r--', 'LineWidth', 2);  % <- 여기만 h로 잡음
% 
% grid on;
% xlabel('time [s]', 'FontWeight', 'bold', 'FontAngle', 'italic', 'FontSize', 16); 
% ylabel('Relative distance [m]', 'FontWeight', 'bold', 'FontAngle', 'italic', 'FontSize', 16);
% xlim([0, 30]); ylim([0 150]);
% set(gca, 'FontSize', 16, ...
%          ...
%          'FontAngle', 'italic', ...
%          'FontName', 'Times New Roman');
% 
% % --- legend: h만 넣기 ---
% legend(h, 'd_{safety}', 'Location', 'best', ...
%     'FontAngle', 'italic', 'FontSize', 16);
% 
% hold off;
timeldx = timeldx + 1;

end

== matlab function ITACG_3D_salvo_simulation/CMMAV1/Guidance/cmd Filter ==
  data: R input; a_y_M input; a_z_M output; a_z_M input; prev_a_y_M input; prev_a_z_M input; a_y_M output
function [a_z_M, a_y_M] = fcn(R, a_y_M, a_z_M, prev_a_y_M, prev_a_z_M)

if R<10
    a_z_M = prev_a_z_M;
    a_y_M = prev_a_y_M;
end

== matlab function ITACG_3D_salvo_simulation/CMMAV4/Guidance/ITACG ==
  data: U output; V input; theta_M input; psi_M input; R input; G input; L input; sigma input; F input; G_inv input
function U  = fcn(V, theta_M, psi_M, R, G, L, sigma, F, G_inv)
    D2R = 180/pi;
    N=4;
    sigma_s = 0.001 * D2R;
    % sigma_deg = sigma*180/pi;
    U_PN = [-sin(psi_M) -sin(theta_M)*cos(psi_M)]';
    %% G_inv
    % U_eq = G_inv * F;

    % if abs(sigma) > sigma_s
    %     U = G_inv * L + U_eq;
    % else
    %     U = N * V^2 * U_PN / R;
    % end
    % U = G_inv * L + U_eq;

    %% G^-1
    U_eq = G^-1 * F;

    if abs(sigma) > sigma_s
        U = G^-1 * L - U_eq;
    else
        U = N * V^2 * U_PN / R;
    end

== matlab function ITACG_3D_salvo_simulation/CMMAV4/Guidance/cmd Filter ==
  data: R input; a_y_M input; a_z_M output; a_z_M input; prev_a_y_M input; prev_a_z_M input; a_y_M output
function [a_z_M, a_y_M] = fcn(R, a_y_M, a_z_M, prev_a_y_M, prev_a_z_M)

if R<10
    a_z_M = prev_a_z_M;
    a_y_M = prev_a_y_M;
end

== matlab function ITACG_3D_salvo_simulation/CMMAV4/Point Mass Model/MATLAB Function ==
  data: LOS_x input; NED_x output; LOS_y input; LOS_z input; psi_L input; theta_L input; NED_y output; NED_z output
function [NED_x, NED_y, NED_z] = fcn(LOS_x, LOS_y, LOS_z, psi_L, theta_L)

% 입력 벡터 (LOS 기준)
v_LOS = [LOS_x; LOS_y; LOS_z];

% 1. LOS → RCS 회전행렬 (T_LOS_to_RCS)
Rz_psi = [cos(psi_L),  sin(psi_L), 0;
         -sin(psi_L),  cos(psi_L), 0;
          0,           0,          1];

Ry_theta = [cos(theta_L), 0, -sin(theta_L);
            0,           1,  0;
            sin(theta_L), 0,  cos(theta_L)];

T_LOS_to_RCS = Ry_theta * Rz_psi;

% 2. RCS → NED 변환 (Z축 반전만 적용)
T_RCS_to_NED = [1, 0,  0;
                0, 1,  0;
                0, 0, -1];

% 전체 변환: LOS → RCS → NED
T_total = T_RCS_to_NED * T_LOS_to_RCS;

v_NED = T_total * v_LOS;

% 결과 추출
NED_x = v_NED(1);
NED_y = v_NED(2);
NED_z = v_NED(3);

end

== matlab function ITACG_3D_salvo_simulation/CMMAV2/Guidance/Geometry ==
  data: V input; theta_M input; psi_M input; R input; R_dot input; G output; L output; t input; t_d input; sigma_max input; psi_L input; theta_L input; theta_LF input; psi_LF input; theta_L_dot input; psi_L_dot input; G_inv output; F output; sigma output; H output; H_dot output; e output; beta output; epsilon_dot output; mu output; mu_dot output
function [G, L, G_inv, F, sigma, H, H_dot, e, beta, epsilon_dot, mu, mu_dot] =fcn(V, theta_M, psi_M, R, R_dot, t, t_d, sigma_max, psi_L, theta_L, theta_LF, psi_LF, theta_L_dot, psi_L_dot)
    %% constant parameter
    b= 0.1;
    k= 1.4;
    eta = 0.5;
    T_s = 0.6 * t_d;

    %% guidance parameter
    sigma = acos(cos(theta_M) * cos(psi_M));
    t_go = t_d - t;

    %% epsilon
    epsilon = t_go - R / V;
    epsilon_dot = cos(sigma) - 1;

    %% theta_e
    theta_e = theta_L - theta_LF;
    theta_e_dot = theta_L_dot;

    %% psi_e
    psi_e = psi_L - psi_LF;
    psi_e_dot = psi_L_dot;

    %% beta
    beta = (theta_e^2 + cos(theta_L)^2 * psi_e^2) / (4 * V^2);
    % beta = sin(sigma)^2 * theta_e / (4 * V^2 * sin(theta_M)^2);

    beta_dot = (theta_e * theta_e_dot + cos(theta_L)^2 * psi_e * psi_e_dot - sin(theta_L) * cos(theta_L) * psi_e^2 * theta_L_dot) / (2 * V^2);

    %% C_f/C_g  
    C_f = psi_e * sin(theta_L) * cos(theta_L);
    C_g = psi_e * cos(theta_M) * cos(theta_L) + theta_e * sin(theta_M) * sin(psi_M);

    %% H
    H = (2 * epsilon^2) / (beta * R^2 + epsilon^2);
    H_dot = ((4 * epsilon * epsilon_dot) / (beta * R^2 + epsilon^2)) - ((2 * epsilon^2 * (beta_dot * R^2 + 2 * beta * R * R_dot + 2 * epsilon * epsilon_dot)) / (beta * R^2 + epsilon^2)^2);
    H_max = 1 - cos(sigma_max);
    H_bar = H / H_max;

    %% chi
    if abs(theta_L) >= pi/2
        chi = theta_e * sin(theta_M);
    else
        chi = psi_e * cos(theta_M) * cos(theta_L) * sin(psi_M) + theta_e * sin(theta_M);
    end
    %% F(H)
    if H < eta * H_max
        f_h = H;
    else
        f_h = ((1 - eta) * tanh((H_bar - eta) / (1 - eta)) + eta) * H_max;
    end
    %% F(H)_dot
    if H < eta * H_max
        f_h_dot = H_dot;
    else
        f_h_dot = (1 - tanh((H_bar - eta) / (1 - eta))^2) * H_dot;
    end

    %% mu    
    if t >= 0 && t < T_s
        mu = T_s / (T_s - t);
        mu_dot = T_s / (T_s - t)^2;
    else
        mu = 1;
        mu_dot = 0;
    end

    %% Baseline Error Dynamics
    % e = [epsilon_dot + H;
    %     psi_e * theta_e_dot - theta_e * psi_e_dot];
    % 
    % F = [-R * theta_L_dot^2 / V - R * psi_L_dot^2 * cos(theta_L)^2 / V + H_dot;
    %     2 * (theta_e * psi_L_dot - psi_e * theta_L_dot) * R_dot / R - C_f * psi_L_dot^2 - 2 * theta_e * psi_L_dot * theta_L_dot * tan(theta_L)]; 

    %% Nonlinear Error Dynamics
    e = [epsilon_dot + f_h;
        psi_e * theta_e_dot - theta_e * psi_e_dot];

    F = [-R * theta_L_dot^2 / V - R * psi_L_dot^2 * cos(theta_L)^2 / V + f_h_dot;
        2 * (theta_e * psi_L_dot - psi_e * theta_L_dot) * R_dot / R - C_f * psi_L_dot^2 - 2 * theta_e * psi_L_dot * theta_L_dot * tan(theta_L)]; 

    %% guidance vector
    G = [-sin(psi_M) / V, -sin(theta_M) * cos(psi_M) / V;
        theta_e * cos(psi_M) / (R * cos(theta_L)), -C_g / (R * cos(theta_L))];

    G_inv = 1 / chi * [-V * C_g, R * sin(theta_M) * cos(psi_M) * cos(theta_L);
        -V * theta_e * cos(psi_M), -R * sin(psi_M) * cos(theta_L)];

    % ne = norm(e);
    L = -(b + k * mu_dot / mu) * e;
